simulink model "T2_DCACpart_solar"  (R2022b)
settings: Solver=VariableStepAuto  StartTime=0.0  StopTime=10.0  RelTol=1e-3
undefined symbols (not defined in the file): High, Low, Ts
libraries: fl_lib x94, nesl_utility x50, simulink x14, ee_lib x2
(part 1 of 2)
settings Model: Creator=mingreico  LastModifiedBy=mingreico

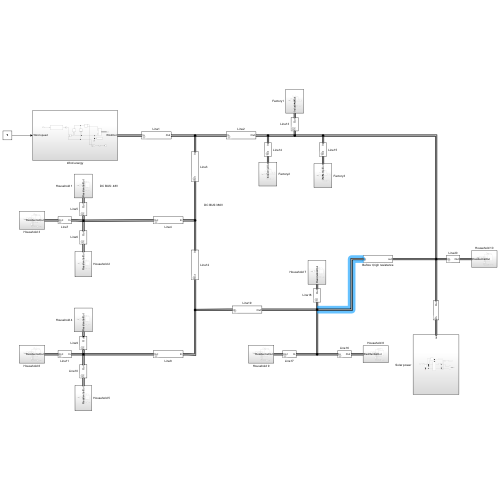
[thumbnail: Simulink's stored preview of the top-level diagram]
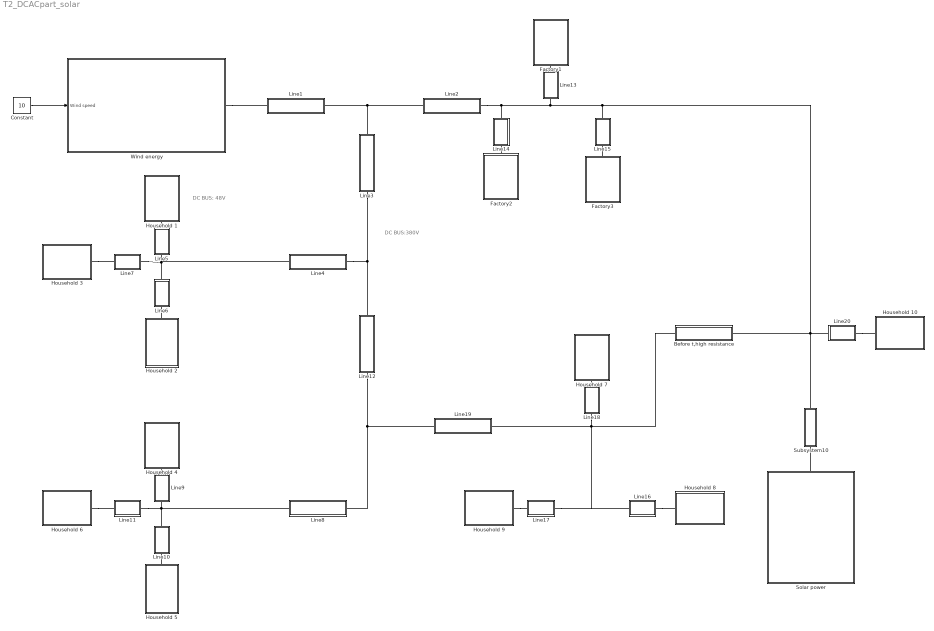
== system T2_DCACpart_solar ==
  note: DC BUS: 48V
  note: DC BUS:380V
  Before t,high resistance : Subsystem  mask{t=48}
      mask prompts: t "Specific jumping time"
  Constant : Constant  Value=10
  Factory1 : Subsystem
  Factory2 : Subsystem
  Factory3 : Subsystem
  Household 1 : Subsystem
  Household 10 : Subsystem
  Household 2 : Subsystem
  Household 3 : Subsystem
  Household 4 : Subsystem
  Household 5 : Subsystem
  Household 6 : Subsystem
  Household 7 : Subsystem
  Household 8 : Subsystem
  Household 9 : Subsystem
  Line1 : Subsystem  mask{rho=1.68e-8, l=2.0, A=1.5e-6}
      mask prompts: rho "Specific resistivity in Ohm*m"; l "Length in m"; A "Cross sectional area in m^2"
  Line10 : Subsystem  mask{rho=1.68e-8, l=2.0, A=1.5e-6}
      mask prompts: rho "Specific resistivity in Ohm*m"; l "Length in m"; A "Cross sectional area in m^2"
  Line11 : Subsystem  mask{rho=1.68e-8, l=2.0, A=1.5e-6}
      mask prompts: rho "Specific resistivity in Ohm*m"; l "Length in m"; A "Cross sectional area in m^2"
  Line12 : Subsystem  mask{rho=1.68e-8, l=2.0, A=1.5e-6}
      mask prompts: rho "Specific resistivity in Ohm*m"; l "Length in m"; A "Cross sectional area in m^2"
  Line13 : Subsystem  mask{rho=1.68e-8, l=2.0, A=1.5e-6}
      mask prompts: rho "Specific resistivity in Ohm*m"; l "Length in m"; A "Cross sectional area in m^2"
  Line14 : Subsystem  mask{rho=1.68e-8, l=2.0, A=1.5e-6}
      mask prompts: rho "Specific resistivity in Ohm*m"; l "Length in m"; A "Cross sectional area in m^2"
  Line15 : Subsystem  mask{rho=1.68e-8, l=2.0, A=1.5e-6}
      mask prompts: rho "Specific resistivity in Ohm*m"; l "Length in m"; A "Cross sectional area in m^2"
  Line16 : Subsystem  mask{rho=1.68e-8, l=2.0, A=1.5e-6}
      mask prompts: rho "Specific resistivity in Ohm*m"; l "Length in m"; A "Cross sectional area in m^2"
  Line17 : Subsystem  mask{rho=1.68e-8, l=2.0, A=1.5e-6}
      mask prompts: rho "Specific resistivity in Ohm*m"; l "Length in m"; A "Cross sectional area in m^2"
  Line18 : Subsystem  mask{rho=1.68e-8, l=2.0, A=1.5e-6}
      mask prompts: rho "Specific resistivity in Ohm*m"; l "Length in m"; A "Cross sectional area in m^2"
  Line19 : Subsystem  mask{rho=1.68e-8, l=2.0, A=1.5e-6}
      mask prompts: rho "Specific resistivity in Ohm*m"; l "Length in m"; A "Cross sectional area in m^2"
  Line2 : Subsystem  mask{rho=1.68e-8, l=2.0, A=1.5e-6}
      mask prompts: rho "Specific resistivity in Ohm*m"; l "Length in m"; A "Cross sectional area in m^2"
  Line20 : Subsystem  mask{rho=1.68e-8, l=2.0, A=1.5e-6}
      mask prompts: rho "Specific resistivity in Ohm*m"; l "Length in m"; A "Cross sectional area in m^2"
  Line3 : Subsystem  mask{rho=1.68e-8, l=2.0, A=1.5e-6}
      mask prompts: rho "Specific resistivity in Ohm*m"; l "Length in m"; A "Cross sectional area in m^2"
  Line4 : Subsystem  mask{rho=1.68e-8, l=2.0, A=1.5e-6}
      mask prompts: rho "Specific resistivity in Ohm*m"; l "Length in m"; A "Cross sectional area in m^2"
  Line5 : Subsystem  mask{rho=1.68e-8, l=2.0, A=1.5e-6}
      mask prompts: rho "Specific resistivity in Ohm*m"; l "Length in m"; A "Cross sectional area in m^2"
  Line6 : Subsystem  mask{rho=1.68e-8, l=2.0, A=1.5e-6}
      mask prompts: rho "Specific resistivity in Ohm*m"; l "Length in m"; A "Cross sectional area in m^2"
  Line7 : Subsystem  mask{rho=1.68e-8, l=2.0, A=1.5e-6}
      mask prompts: rho "Specific resistivity in Ohm*m"; l "Length in m"; A "Cross sectional area in m^2"
  Line8 : Subsystem  mask{rho=1.68e-8, l=2.0, A=1.5e-6}
      mask prompts: rho "Specific resistivity in Ohm*m"; l "Length in m"; A "Cross sectional area in m^2"
  Line9 : Subsystem  mask{rho=1.68e-8, l=2.0, A=1.5e-6}
      mask prompts: rho "Specific resistivity in Ohm*m"; l "Length in m"; A "Cross sectional area in m^2"
  Solar power : Subsystem
  Subsystem10 : Subsystem  mask{rho=1.68e-8, l=2.0, A=1.5e-6}
      mask prompts: rho "Specific resistivity in Ohm*m"; l "Length in m"; A "Cross sectional area in m^2"
  Wind energy : Subsystem
  wires:
  Constant/1 -> Wind energy/1(Wind speed)
  connections:
  Wind energy/RConn1 -- Line1/LConn1
  Line2/LConn1 -- Line3/LConn1 -- Line1/RConn1
  Household 1/RConn1 -- Line5/RConn1
  Household 3/RConn1 -- Line7/RConn1
  Household 2/RConn1 -- Line6/LConn1
  Line5/LConn1 -- Line6/RConn1 -- Line7/LConn1 -- Line4/RConn1
  Line9/LConn1 -- Line11/LConn1 -- Line10/RConn1 -- Line8/RConn1
  Household 5/RConn1 -- Line10/LConn1
  Household 6/RConn1 -- Line11/RConn1
  Household 4/RConn1 -- Line9/RConn1
  Line3/RConn1 -- Line4/LConn1 -- Line12/LConn1
  Line12/RConn1 -- Line19/LConn1 -- Line8/LConn1
  Line2/RConn1 -- Line14/LConn1 -- Line13/LConn1 -- Before t,high resistance/RConn1 -- Line20/LConn1 -- Subsystem10/RConn1 -- Line15/LConn1
  Factory1/RConn1 -- Line13/RConn1
  Factory2/RConn1 -- Line14/RConn1
  Factory3/RConn1 -- Line15/RConn1
  Household 9/RConn1 -- Line17/RConn1
  Household 7/RConn1 -- Line18/RConn1
  Line18/LConn1 -- Before t,high resistance/LConn1 -- Line16/LConn1 -- Line17/LConn1 -- Line19/RConn1
  Line16/RConn1 -- Household 8/RConn1
  Line20/RConn1 -- Household 10/RConn1
  Solar power/LConn1 -- Subsystem10/LConn1

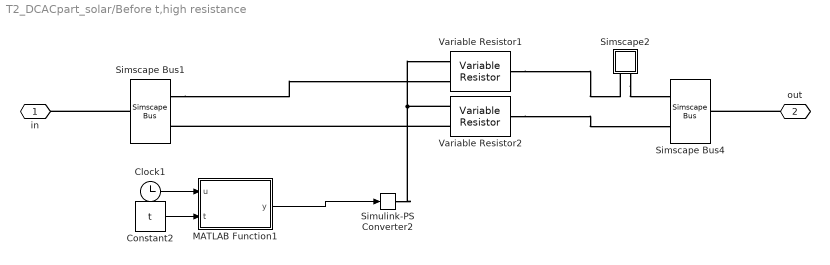
== system T2_DCACpart_solar/Before t,high resistance ==
  Clock1 : Clock
  Constant2 : Constant  Value=t
  MATLAB Function1 : MATLAB Function  TreatAsAtomicUnit=on
  Simscape Bus1 : SimscapeBus  HierarchyStrings=High;Low
  Simscape Bus4 : SimscapeBus  HierarchyStrings=High;Low
  Simscape2 : Subsystem
      mask Display:
      | disp('A')
      | port_label('LConn',1,'+')
      | port_label('LConn',2,'-')
  Simulink-PS Converter2 : nesl_utility/Simulink-PS Converter  PhysicalDomain=network_engine_domain  SubClassName=ps_input  LeftPortType=input  RightPortType=output  PseudoPeriodic=off  Frequencies=[]  NoiseDistribution=none  NoiseParameters=[]  Unit=1  AffineConversion=off  FilteringAndDerivatives=provide  SimscapeFilterOrder=1  InputFilterTimeConstant=0.001  UdotUserProvided=0
  Variable Resistor1 : fl_lib/Electrical/Electrical Elements/Variable Resistor  Rmin=0 Ohm  i_specify=off  i_priority=None  i=0 A  i_nominal_specify=off  i_nominal_unit=A  i_nominal_value=1  v_specify=off  v_priority=None  v=0 V  v_nominal_specify=off  v_nominal_unit=V  v_nominal_value=1
  Variable Resistor2 : fl_lib/Electrical/Electrical Elements/Variable Resistor  Rmin=0 Ohm  i_specify=off  i_priority=None  i=0 A  i_nominal_specify=off  i_nominal_unit=A  i_nominal_value=1  v_specify=off  v_priority=None  v=0 V  v_nominal_specify=off  v_nominal_unit=V  v_nominal_value=1
  in : PMIOPort  Side=Left
  out : PMIOPort  Port=2  Side=Right
  wires:
  MATLAB Function1/1(y) -> Simulink-PS Converter2/1
  Constant2/1 -> MATLAB Function1/2(t)
  Clock1/1 -> MATLAB Function1/1(u)
  connections:
  out/RConn1 -- Simscape Bus4/RConn1
  Simscape Bus1/RConn1 -- in/RConn1
  Variable Resistor2/LConn2 -- Simscape Bus1/LConn2
  Simscape Bus1/LConn1 -- Variable Resistor1/LConn2
  Variable Resistor1/RConn1 -- Simscape2/LConn1
  Variable Resistor2/RConn1 -- Simscape Bus4/LConn2
  Simulink-PS Converter2/RConn1 -- Variable Resistor2/LConn1 -- Variable Resistor1/LConn1
  Simscape2/LConn2 -- Simscape Bus4/LConn1

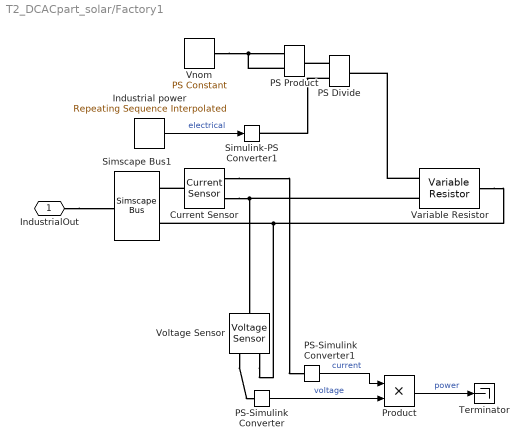
== system T2_DCACpart_solar/Factory1 ==
  Current Sensor : fl_lib/Electrical/Electrical Sensors/Current Sensor
  "Industrial power " : simulink/Sources/Repeating Sequence Interpolated  OutValues=[6.0 5.9 5.9 5.9 5.8 5.7 5.6 5.5 5.7 5.9 5.9 5.3 5.3 5.6 5.9 5.8 5.6 5.3 5.3 5.7 5.9 5.9 6.0 6.0]*1000  TimeValues=[0 1 2 3 4 5 6 7 8 9 10 11 12 13 14 15 16 17 18 19 20 21 22 23]  LookUpMeth=Interpolation-Use End Values  tsamp=1e-4  OutMin=[]  OutMax=[]  OutDataTypeStr=double  OutputDataTypeScalingMode=double  OutDataType=fixdt(0,8)  OutScaling=2^-10
  PS Divide : fl_lib/Physical Signals/Functions/PS Divide
  PS Product : fl_lib/Physical Signals/Functions/PS Product
  PS-Simulink Converter : nesl_utility/PS-Simulink Converter  PhysicalDomain=network_engine_domain  SubClassName=ps_output  LeftPortType=input  RightPortType=output  PseudoPeriodic=off  Frequencies=[]  VectorFormat=inherit  Unit=inherit  AffineConversion=off
  PS-Simulink Converter1 : nesl_utility/PS-Simulink Converter  PhysicalDomain=network_engine_domain  SubClassName=ps_output  LeftPortType=input  RightPortType=output  PseudoPeriodic=off  Frequencies=[]  VectorFormat=inherit  Unit=inherit  AffineConversion=off
  Product : Product
  Simscape Bus1 : SimscapeBus  HierarchyStrings=High;Low
  Simulink-PS Converter1 : nesl_utility/Simulink-PS Converter  PhysicalDomain=network_engine_domain  SubClassName=ps_input  LeftPortType=input  RightPortType=output  PseudoPeriodic=off  Frequencies=[]  NoiseDistribution=none  NoiseParameters=[]  Unit=V*A  AffineConversion=off  FilteringAndDerivatives=provide  SimscapeFilterOrder=1  InputFilterTimeConstant=0.001  UdotUserProvided=0
  Terminator : Terminator
  Variable Resistor : fl_lib/Electrical/Electrical Elements/Variable Resistor  Rmin=0 Ohm  i_specify=off  i_priority=None  i=0 A  i_nominal_specify=off  i_nominal_unit=A  i_nominal_value=1  v_specify=off  v_priority=None  v=0 V  v_nominal_specify=off  v_nominal_unit=V  v_nominal_value=1
  Vnom : fl_lib/Physical Signals/Sources/PS Constant  constant=48 V
  Voltage Sensor : fl_lib/Electrical/Electrical Sensors/Voltage Sensor
  IndustrialOut : PMIOPort  Side=Right
  wires:
  Product/1 -> Terminator/1  "power"
  PS-Simulink Converter1/1 -> Product/1  "current"
  PS-Simulink Converter/1 -> Product/2  "voltage"
  "Industrial power "/1 -> Simulink-PS Converter1/1  "electrical"
  connections:
  Current Sensor/RConn1 -- PS-Simulink Converter1/LConn1
  Current Sensor/LConn1 -- Simscape Bus1/LConn1
  Voltage Sensor/RConn1 -- PS-Simulink Converter/LConn1
  Current Sensor/RConn2 -- Variable Resistor/LConn2 -- Voltage Sensor/LConn1
  IndustrialOut/RConn1 -- Simscape Bus1/RConn1
  Voltage Sensor/RConn2 -- Simscape Bus1/LConn2 -- Variable Resistor/RConn1
  Vnom/RConn1 -- PS Product/LConn2 -- PS Product/LConn1
  PS Divide/LConn2 -- Simulink-PS Converter1/RConn1
  Variable Resistor/LConn1 -- PS Divide/RConn1
  PS Divide/LConn1 -- PS Product/RConn1

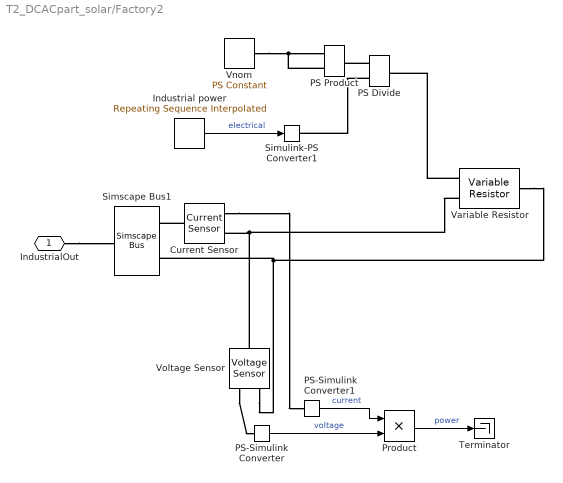
== system T2_DCACpart_solar/Factory2 ==
  Current Sensor : fl_lib/Electrical/Electrical Sensors/Current Sensor
  "Industrial power " : simulink/Sources/Repeating Sequence Interpolated  OutValues=[6.0 5.9 5.9 5.9 5.8 5.7 5.6 5.5 5.7 5.9 5.9 5.3 5.3 5.6 5.9 5.8 5.6 5.3 5.3 5.7 5.9 5.9 6.0 6.0]*1000  TimeValues=[0 1 2 3 4 5 6 7 8 9 10 11 12 13 14 15 16 17 18 19 20 21 22 23]  LookUpMeth=Interpolation-Use End Values  tsamp=1e-4  OutMin=[]  OutMax=[]  OutDataTypeStr=double  OutputDataTypeScalingMode=double  OutDataType=fixdt(0,8)  OutScaling=2^-10
  PS Divide : fl_lib/Physical Signals/Functions/PS Divide
  PS Product : fl_lib/Physical Signals/Functions/PS Product
  PS-Simulink Converter : nesl_utility/PS-Simulink Converter  PhysicalDomain=network_engine_domain  SubClassName=ps_output  LeftPortType=input  RightPortType=output  PseudoPeriodic=off  Frequencies=[]  VectorFormat=inherit  Unit=inherit  AffineConversion=off
  PS-Simulink Converter1 : nesl_utility/PS-Simulink Converter  PhysicalDomain=network_engine_domain  SubClassName=ps_output  LeftPortType=input  RightPortType=output  PseudoPeriodic=off  Frequencies=[]  VectorFormat=inherit  Unit=inherit  AffineConversion=off
  Product : Product
  Simscape Bus1 : SimscapeBus  HierarchyStrings=High;Low
  Simulink-PS Converter1 : nesl_utility/Simulink-PS Converter  PhysicalDomain=network_engine_domain  SubClassName=ps_input  LeftPortType=input  RightPortType=output  PseudoPeriodic=off  Frequencies=[]  NoiseDistribution=none  NoiseParameters=[]  Unit=V*A  AffineConversion=off  FilteringAndDerivatives=provide  SimscapeFilterOrder=1  InputFilterTimeConstant=0.001  UdotUserProvided=0
  Terminator : Terminator
  Variable Resistor : fl_lib/Electrical/Electrical Elements/Variable Resistor  Rmin=0 Ohm  i_specify=off  i_priority=None  i=0 A  i_nominal_specify=off  i_nominal_unit=A  i_nominal_value=1  v_specify=off  v_priority=None  v=0 V  v_nominal_specify=off  v_nominal_unit=V  v_nominal_value=1
  Vnom : fl_lib/Physical Signals/Sources/PS Constant  constant=48 V
  Voltage Sensor : fl_lib/Electrical/Electrical Sensors/Voltage Sensor
  IndustrialOut : PMIOPort  Side=Right
  wires:
  PS-Simulink Converter/1 -> Product/2  "voltage"
  PS-Simulink Converter1/1 -> Product/1  "current"
  Product/1 -> Terminator/1  "power"
  "Industrial power "/1 -> Simulink-PS Converter1/1  "electrical"
  connections:
  Voltage Sensor/RConn2 -- Variable Resistor/RConn1 -- Simscape Bus1/LConn2
  IndustrialOut/RConn1 -- Simscape Bus1/RConn1
  Voltage Sensor/LConn1 -- Variable Resistor/LConn2 -- Current Sensor/RConn2
  Voltage Sensor/RConn1 -- PS-Simulink Converter/LConn1
  Current Sensor/LConn1 -- Simscape Bus1/LConn1
  Current Sensor/RConn1 -- PS-Simulink Converter1/LConn1
  Vnom/RConn1 -- PS Product/LConn2 -- PS Product/LConn1
  Variable Resistor/LConn1 -- PS Divide/RConn1
  PS Divide/LConn1 -- PS Product/RConn1
  PS Divide/LConn2 -- Simulink-PS Converter1/RConn1

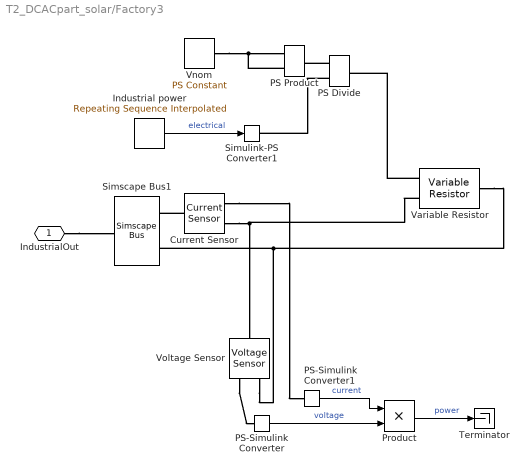
== system T2_DCACpart_solar/Factory3 ==
  Current Sensor : fl_lib/Electrical/Electrical Sensors/Current Sensor
  "Industrial power " : simulink/Sources/Repeating Sequence Interpolated  OutValues=[6.0 5.9 5.9 5.9 5.8 5.7 5.6 5.5 5.7 5.9 5.9 5.3 5.3 5.6 5.9 5.8 5.6 5.3 5.3 5.7 5.9 5.9 6.0 6.0]*1000  TimeValues=[0 1 2 3 4 5 6 7 8 9 10 11 12 13 14 15 16 17 18 19 20 21 22 23]  LookUpMeth=Interpolation-Use End Values  tsamp=1e-4  OutMin=[]  OutMax=[]  OutDataTypeStr=double  OutputDataTypeScalingMode=double  OutDataType=fixdt(0,8)  OutScaling=2^-10
  PS Divide : fl_lib/Physical Signals/Functions/PS Divide
  PS Product : fl_lib/Physical Signals/Functions/PS Product
  PS-Simulink Converter : nesl_utility/PS-Simulink Converter  PhysicalDomain=network_engine_domain  SubClassName=ps_output  LeftPortType=input  RightPortType=output  PseudoPeriodic=off  Frequencies=[]  VectorFormat=inherit  Unit=inherit  AffineConversion=off
  PS-Simulink Converter1 : nesl_utility/PS-Simulink Converter  PhysicalDomain=network_engine_domain  SubClassName=ps_output  LeftPortType=input  RightPortType=output  PseudoPeriodic=off  Frequencies=[]  VectorFormat=inherit  Unit=inherit  AffineConversion=off
  Product : Product
  Simscape Bus1 : SimscapeBus  HierarchyStrings=High;Low
  Simulink-PS Converter1 : nesl_utility/Simulink-PS Converter  PhysicalDomain=network_engine_domain  SubClassName=ps_input  LeftPortType=input  RightPortType=output  PseudoPeriodic=off  Frequencies=[]  NoiseDistribution=none  NoiseParameters=[]  Unit=V*A  AffineConversion=off  FilteringAndDerivatives=provide  SimscapeFilterOrder=1  InputFilterTimeConstant=0.001  UdotUserProvided=0
  Terminator : Terminator
  Variable Resistor : fl_lib/Electrical/Electrical Elements/Variable Resistor  Rmin=0 Ohm  i_specify=off  i_priority=None  i=0 A  i_nominal_specify=off  i_nominal_unit=A  i_nominal_value=1  v_specify=off  v_priority=None  v=0 V  v_nominal_specify=off  v_nominal_unit=V  v_nominal_value=1
  Vnom : fl_lib/Physical Signals/Sources/PS Constant  constant=48 V
  Voltage Sensor : fl_lib/Electrical/Electrical Sensors/Voltage Sensor
  IndustrialOut : PMIOPort  Side=Right
  wires:
  Product/1 -> Terminator/1  "power"
  PS-Simulink Converter1/1 -> Product/1  "current"
  PS-Simulink Converter/1 -> Product/2  "voltage"
  "Industrial power "/1 -> Simulink-PS Converter1/1  "electrical"
  connections:
  Current Sensor/RConn1 -- PS-Simulink Converter1/LConn1
  Current Sensor/LConn1 -- Simscape Bus1/LConn1
  Voltage Sensor/RConn1 -- PS-Simulink Converter/LConn1
  Current Sensor/RConn2 -- Variable Resistor/LConn2 -- Voltage Sensor/LConn1
  IndustrialOut/RConn1 -- Simscape Bus1/RConn1
  Voltage Sensor/RConn2 -- Simscape Bus1/LConn2 -- Variable Resistor/RConn1
  Vnom/RConn1 -- PS Product/LConn2 -- PS Product/LConn1
  Variable Resistor/LConn1 -- PS Divide/RConn1
  PS Divide/LConn1 -- PS Product/RConn1
  PS Divide/LConn2 -- Simulink-PS Converter1/RConn1

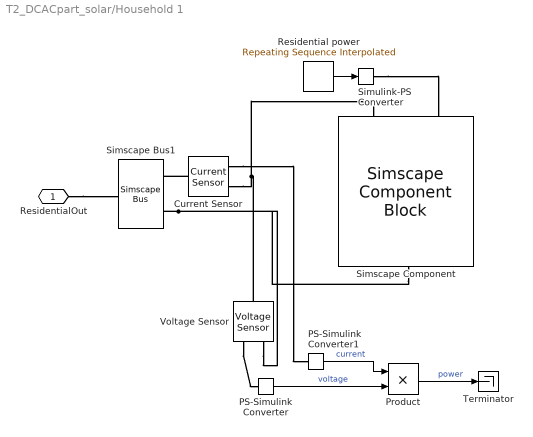
== system T2_DCACpart_solar/Household 1 ==
  Current Sensor : fl_lib/Electrical/Electrical Sensors/Current Sensor
  PS-Simulink Converter : nesl_utility/PS-Simulink Converter  PhysicalDomain=network_engine_domain  SubClassName=ps_output  LeftPortType=input  RightPortType=output  PseudoPeriodic=off  Frequencies=[]  VectorFormat=inherit  Unit=inherit  AffineConversion=off
  PS-Simulink Converter1 : nesl_utility/PS-Simulink Converter  PhysicalDomain=network_engine_domain  SubClassName=ps_output  LeftPortType=input  RightPortType=output  PseudoPeriodic=off  Frequencies=[]  VectorFormat=inherit  Unit=inherit  AffineConversion=off
  Product : Product
  "Residential power " : simulink/Sources/Repeating Sequence Interpolated  OutValues=[2.8 2.5 2 2 2.2 2.5 2.8 3.4 3.6 3.8 4 4 4 4 4 4 4 4 4 4 3.8 3.5 3.2 3]*1000  TimeValues=[0 1 2 3 4 5 6 7 8 9 10 11 12 13 14 15 16 17 18 19 20 21 22 23]  LookUpMeth=Interpolation-Use End Values  tsamp=1e-4  OutMin=[]  OutMax=[]  OutDataTypeStr=double  OutputDataTypeScalingMode=double  OutDataType=fixdt(0,8)  OutScaling=2^-10
  Simscape Component : SimscapeComponentBlock  SourceFile=ResidentialPowerLoad  ComponentPath=ResidentialPowerLoad  ComponentVariants="[\"ResidentialPowerLoad\"]"  ComponentVariantNames="[\"ResidentialPowerLoad\"]"  ClassName=ResidentialPowerLoad  SchemaVersion=1  i_specify=off  i_priority=None  i=0 A  i_nominal_specify=off  i_nominal_unit=A  i_nominal_value=1  v_specify=off  v_priority=None  v=0 V  v_nominal_specify=off  v_nominal_unit=V  v_nominal_value=1
      settings: CopyFcn=simscape.engine.sli.internal.componentblockcallback(gcbh,'COPY')  PreCopyFcn=simscape.engine.sli.internal.componentblockcallback(gcbh,'PRECOPY')  PreDeleteFcn=simscape.engine.sli.internal.componentblockcallback(gcbh,'PREDELETE')  InternalSimscapePortConfiguration="{\"Bottom\":[],\"Left\":[{\"id\":\"Power\",\"label\":\"P\",\"type\":\"input\"},{\"id\":\"p\",\"label\":\"+\",\"type\":\"foundation.electrical.electrical\"}],\"Right\":[{\"id\":\"n\",\"label\":\"-\",\"type\":\"foundation.electrical.electrical\"}],\"Top\":[]}"
      mask Type: ResidentialPowerLoad
      mask Display: color('red');plot([0 1 1 0 0],[0 0 1 1 0]);plot([0.7,1],[1,0.7]);plot(-2,-1.75);plot(3, 1);disp('\n.ssc\nUnresolved')
  Simscape Bus1 : SimscapeBus  HierarchyStrings=High;Low
  Simulink-PS Converter : nesl_utility/Simulink-PS Converter  PhysicalDomain=network_engine_domain  SubClassName=ps_input  LeftPortType=input  RightPortType=output  PseudoPeriodic=off  Frequencies=[]  NoiseDistribution=none  NoiseParameters=[]  Unit=1  AffineConversion=off  FilteringAndDerivatives=provide  SimscapeFilterOrder=1  InputFilterTimeConstant=0.001  UdotUserProvided=0
  Terminator : Terminator
  Voltage Sensor : fl_lib/Electrical/Electrical Sensors/Voltage Sensor
  ResidentialOut : PMIOPort  Side=Right
  wires:
  "Residential power "/1 -> Simulink-PS Converter/1
  PS-Simulink Converter/1 -> Product/2  "voltage"
  PS-Simulink Converter1/1 -> Product/1  "current"
  Product/1 -> Terminator/1  "power"
  connections:
  Simscape Bus1/LConn2 -- Simscape Component/RConn1 -- Voltage Sensor/RConn2
  ResidentialOut/RConn1 -- Simscape Bus1/RConn1
  Current Sensor/RConn2 -- Voltage Sensor/LConn1 -- Simscape Component/LConn2
  Voltage Sensor/RConn1 -- PS-Simulink Converter/LConn1
  Simulink-PS Converter/RConn1 -- Simscape Component/LConn1
  Current Sensor/LConn1 -- Simscape Bus1/LConn1
  Current Sensor/RConn1 -- PS-Simulink Converter1/LConn1

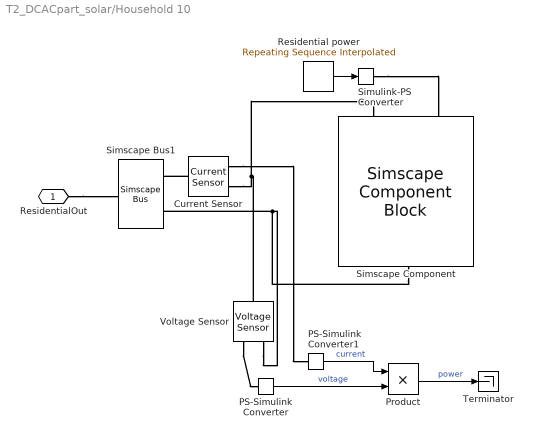
== system T2_DCACpart_solar/Household 10 ==
  Current Sensor : fl_lib/Electrical/Electrical Sensors/Current Sensor
  PS-Simulink Converter : nesl_utility/PS-Simulink Converter  PhysicalDomain=network_engine_domain  SubClassName=ps_output  LeftPortType=input  RightPortType=output  PseudoPeriodic=off  Frequencies=[]  VectorFormat=inherit  Unit=inherit  AffineConversion=off
  PS-Simulink Converter1 : nesl_utility/PS-Simulink Converter  PhysicalDomain=network_engine_domain  SubClassName=ps_output  LeftPortType=input  RightPortType=output  PseudoPeriodic=off  Frequencies=[]  VectorFormat=inherit  Unit=inherit  AffineConversion=off
  Product : Product
  "Residential power " : simulink/Sources/Repeating Sequence Interpolated  OutValues=[2.8 2.5 2 2 2.2 2.5 2.8 3.4 3.6 3.8 4 4 4 4 4 4 4 4 4 4 3.8 3.5 3.2 3]*1000  TimeValues=[0 1 2 3 4 5 6 7 8 9 10 11 12 13 14 15 16 17 18 19 20 21 22 23]  LookUpMeth=Interpolation-Use End Values  tsamp=1e-4  OutMin=[]  OutMax=[]  OutDataTypeStr=double  OutputDataTypeScalingMode=double  OutDataType=fixdt(0,8)  OutScaling=2^-10
  Simscape Component : SimscapeComponentBlock  SourceFile=ResidentialPowerLoad  ComponentPath=ResidentialPowerLoad  ComponentVariants="[\"ResidentialPowerLoad\"]"  ComponentVariantNames="[\"ResidentialPowerLoad\"]"  ClassName=ResidentialPowerLoad  SchemaVersion=1  i_specify=off  i_priority=None  i=0 A  i_nominal_specify=off  i_nominal_unit=A  i_nominal_value=1  v_specify=off  v_priority=None  v=0 V  v_nominal_specify=off  v_nominal_unit=V  v_nominal_value=1
      settings: CopyFcn=simscape.engine.sli.internal.componentblockcallback(gcbh,'COPY')  PreCopyFcn=simscape.engine.sli.internal.componentblockcallback(gcbh,'PRECOPY')  PreDeleteFcn=simscape.engine.sli.internal.componentblockcallback(gcbh,'PREDELETE')  InternalSimscapePortConfiguration="{\"Bottom\":[],\"Left\":[{\"id\":\"Power\",\"label\":\"P\",\"type\":\"input\"},{\"id\":\"p\",\"label\":\"+\",\"type\":\"foundation.electrical.electrical\"}],\"Right\":[{\"id\":\"n\",\"label\":\"-\",\"type\":\"foundation.electrical.electrical\"}],\"Top\":[]}"
      mask Type: ResidentialPowerLoad
      mask Display: color('red');plot([0 1 1 0 0],[0 0 1 1 0]);plot([0.7,1],[1,0.7]);plot(-2,-1.75);plot(3, 1);disp('\n.ssc\nUnresolved')
  Simscape Bus1 : SimscapeBus  HierarchyStrings=High;Low
  Simulink-PS Converter : nesl_utility/Simulink-PS Converter  PhysicalDomain=network_engine_domain  SubClassName=ps_input  LeftPortType=input  RightPortType=output  PseudoPeriodic=off  Frequencies=[]  NoiseDistribution=none  NoiseParameters=[]  Unit=1  AffineConversion=off  FilteringAndDerivatives=provide  SimscapeFilterOrder=1  InputFilterTimeConstant=0.001  UdotUserProvided=0
  Terminator : Terminator
  Voltage Sensor : fl_lib/Electrical/Electrical Sensors/Voltage Sensor
  ResidentialOut : PMIOPort  Side=Right
  wires:
  Product/1 -> Terminator/1  "power"
  PS-Simulink Converter1/1 -> Product/1  "current"
  PS-Simulink Converter/1 -> Product/2  "voltage"
  "Residential power "/1 -> Simulink-PS Converter/1
  connections:
  Current Sensor/RConn1 -- PS-Simulink Converter1/LConn1
  Current Sensor/LConn1 -- Simscape Bus1/LConn1
  Simulink-PS Converter/RConn1 -- Simscape Component/LConn1
  Voltage Sensor/RConn1 -- PS-Simulink Converter/LConn1
  Voltage Sensor/LConn1 -- Current Sensor/RConn2 -- Simscape Component/LConn2
  ResidentialOut/RConn1 -- Simscape Bus1/RConn1
  Simscape Component/RConn1 -- Simscape Bus1/LConn2 -- Voltage Sensor/RConn2

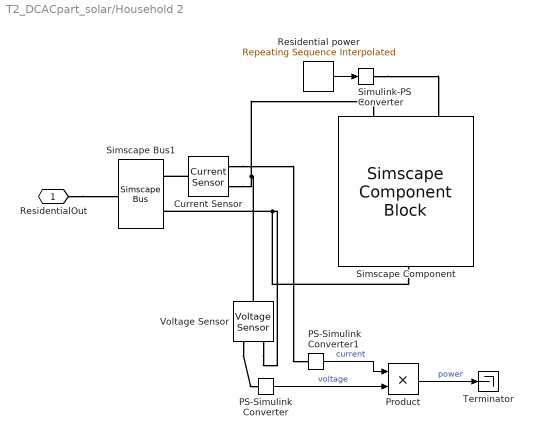
== system T2_DCACpart_solar/Household 2 ==
  Current Sensor : fl_lib/Electrical/Electrical Sensors/Current Sensor
  PS-Simulink Converter : nesl_utility/PS-Simulink Converter  PhysicalDomain=network_engine_domain  SubClassName=ps_output  LeftPortType=input  RightPortType=output  PseudoPeriodic=off  Frequencies=[]  VectorFormat=inherit  Unit=inherit  AffineConversion=off
  PS-Simulink Converter1 : nesl_utility/PS-Simulink Converter  PhysicalDomain=network_engine_domain  SubClassName=ps_output  LeftPortType=input  RightPortType=output  PseudoPeriodic=off  Frequencies=[]  VectorFormat=inherit  Unit=inherit  AffineConversion=off
  Product : Product
  "Residential power " : simulink/Sources/Repeating Sequence Interpolated  OutValues=[2.8 2.5 2 2 2.2 2.5 2.8 3.4 3.6 3.8 4 4 4 4 4 4 4 4 4 4 3.8 3.5 3.2 3]*1000  TimeValues=[0 1 2 3 4 5 6 7 8 9 10 11 12 13 14 15 16 17 18 19 20 21 22 23]  LookUpMeth=Interpolation-Use End Values  tsamp=1e-4  OutMin=[]  OutMax=[]  OutDataTypeStr=double  OutputDataTypeScalingMode=double  OutDataType=fixdt(0,8)  OutScaling=2^-10
  Simscape Component : SimscapeComponentBlock  SourceFile=ResidentialPowerLoad  ComponentPath=ResidentialPowerLoad  ComponentVariants="[\"ResidentialPowerLoad\"]"  ComponentVariantNames="[\"ResidentialPowerLoad\"]"  ClassName=ResidentialPowerLoad  SchemaVersion=1  i_specify=off  i_priority=None  i=0 A  i_nominal_specify=off  i_nominal_unit=A  i_nominal_value=1  v_specify=off  v_priority=None  v=0 V  v_nominal_specify=off  v_nominal_unit=V  v_nominal_value=1
      settings: CopyFcn=simscape.engine.sli.internal.componentblockcallback(gcbh,'COPY')  PreCopyFcn=simscape.engine.sli.internal.componentblockcallback(gcbh,'PRECOPY')  PreDeleteFcn=simscape.engine.sli.internal.componentblockcallback(gcbh,'PREDELETE')  InternalSimscapePortConfiguration="{\"Bottom\":[],\"Left\":[{\"id\":\"Power\",\"label\":\"P\",\"type\":\"input\"},{\"id\":\"p\",\"label\":\"+\",\"type\":\"foundation.electrical.electrical\"}],\"Right\":[{\"id\":\"n\",\"label\":\"-\",\"type\":\"foundation.electrical.electrical\"}],\"Top\":[]}"
      mask Type: ResidentialPowerLoad
      mask Display: color('red');plot([0 1 1 0 0],[0 0 1 1 0]);plot([0.7,1],[1,0.7]);plot(-2,-1.75);plot(3, 1);disp('\n.ssc\nUnresolved')
  Simscape Bus1 : SimscapeBus  HierarchyStrings=High;Low
  Simulink-PS Converter : nesl_utility/Simulink-PS Converter  PhysicalDomain=network_engine_domain  SubClassName=ps_input  LeftPortType=input  RightPortType=output  PseudoPeriodic=off  Frequencies=[]  NoiseDistribution=none  NoiseParameters=[]  Unit=1  AffineConversion=off  FilteringAndDerivatives=provide  SimscapeFilterOrder=1  InputFilterTimeConstant=0.001  UdotUserProvided=0
  Terminator : Terminator
  Voltage Sensor : fl_lib/Electrical/Electrical Sensors/Voltage Sensor
  ResidentialOut : PMIOPort  Side=Right
  wires:
  Product/1 -> Terminator/1  "power"
  PS-Simulink Converter1/1 -> Product/1  "current"
  PS-Simulink Converter/1 -> Product/2  "voltage"
  "Residential power "/1 -> Simulink-PS Converter/1
  connections:
  Current Sensor/RConn1 -- PS-Simulink Converter1/LConn1
  Current Sensor/LConn1 -- Simscape Bus1/LConn1
  Simulink-PS Converter/RConn1 -- Simscape Component/LConn1
  Voltage Sensor/RConn1 -- PS-Simulink Converter/LConn1
  Voltage Sensor/LConn1 -- Current Sensor/RConn2 -- Simscape Component/LConn2
  ResidentialOut/RConn1 -- Simscape Bus1/RConn1
  Simscape Component/RConn1 -- Simscape Bus1/LConn2 -- Voltage Sensor/RConn2

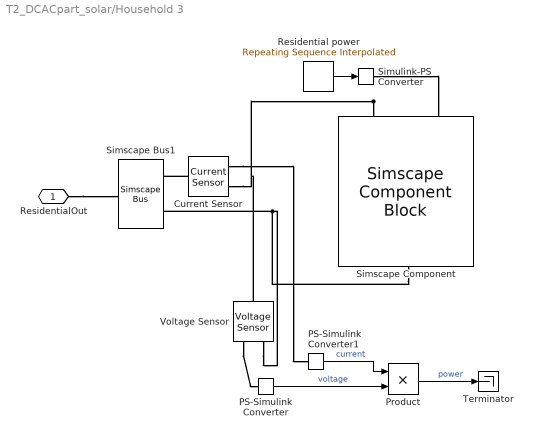
== system T2_DCACpart_solar/Household 3 ==
  Current Sensor : fl_lib/Electrical/Electrical Sensors/Current Sensor
  PS-Simulink Converter : nesl_utility/PS-Simulink Converter  PhysicalDomain=network_engine_domain  SubClassName=ps_output  LeftPortType=input  RightPortType=output  PseudoPeriodic=off  Frequencies=[]  VectorFormat=inherit  Unit=inherit  AffineConversion=off
  PS-Simulink Converter1 : nesl_utility/PS-Simulink Converter  PhysicalDomain=network_engine_domain  SubClassName=ps_output  LeftPortType=input  RightPortType=output  PseudoPeriodic=off  Frequencies=[]  VectorFormat=inherit  Unit=inherit  AffineConversion=off
  Product : Product
  "Residential power " : simulink/Sources/Repeating Sequence Interpolated  OutValues=[2.8 2.5 2 2 2.2 2.5 2.8 3.4 3.6 3.8 4 4 4 4 4 4 4 4 4 4 3.8 3.5 3.2 3]*1000  TimeValues=[0 1 2 3 4 5 6 7 8 9 10 11 12 13 14 15 16 17 18 19 20 21 22 23]  LookUpMeth=Interpolation-Use End Values  tsamp=1e-4  OutMin=[]  OutMax=[]  OutDataTypeStr=double  OutputDataTypeScalingMode=double  OutDataType=fixdt(0,8)  OutScaling=2^-10
  Simscape Component : SimscapeComponentBlock  SourceFile=ResidentialPowerLoad  ComponentPath=ResidentialPowerLoad  ComponentVariants="[\"ResidentialPowerLoad\"]"  ComponentVariantNames="[\"ResidentialPowerLoad\"]"  ClassName=ResidentialPowerLoad  SchemaVersion=1  i_specify=off  i_priority=None  i=0 A  i_nominal_specify=off  i_nominal_unit=A  i_nominal_value=1  v_specify=off  v_priority=None  v=0 V  v_nominal_specify=off  v_nominal_unit=V  v_nominal_value=1
      settings: CopyFcn=simscape.engine.sli.internal.componentblockcallback(gcbh,'COPY')  PreCopyFcn=simscape.engine.sli.internal.componentblockcallback(gcbh,'PRECOPY')  PreDeleteFcn=simscape.engine.sli.internal.componentblockcallback(gcbh,'PREDELETE')  InternalSimscapePortConfiguration="{\"Bottom\":[],\"Left\":[{\"id\":\"Power\",\"label\":\"P\",\"type\":\"input\"},{\"id\":\"p\",\"label\":\"+\",\"type\":\"foundation.electrical.electrical\"}],\"Right\":[{\"id\":\"n\",\"label\":\"-\",\"type\":\"foundation.electrical.electrical\"}],\"Top\":[]}"
      mask Type: ResidentialPowerLoad
      mask Display: color('red');plot([0 1 1 0 0],[0 0 1 1 0]);plot([0.7,1],[1,0.7]);plot(-2,-1.75);plot(3, 1);disp('\n.ssc\nUnresolved')
  Simscape Bus1 : SimscapeBus  HierarchyStrings=High;Low
  Simulink-PS Converter : nesl_utility/Simulink-PS Converter  PhysicalDomain=network_engine_domain  SubClassName=ps_input  LeftPortType=input  RightPortType=output  PseudoPeriodic=off  Frequencies=[]  NoiseDistribution=none  NoiseParameters=[]  Unit=1  AffineConversion=off  FilteringAndDerivatives=provide  SimscapeFilterOrder=1  InputFilterTimeConstant=0.001  UdotUserProvided=0
  Terminator : Terminator
  Voltage Sensor : fl_lib/Electrical/Electrical Sensors/Voltage Sensor
  ResidentialOut : PMIOPort  Side=Right
  wires:
  "Residential power "/1 -> Simulink-PS Converter/1
  PS-Simulink Converter/1 -> Product/2  "voltage"
  PS-Simulink Converter1/1 -> Product/1  "current"
  Product/1 -> Terminator/1  "power"
  connections:
  Voltage Sensor/RConn2 -- Simscape Bus1/LConn2 -- Simscape Component/RConn1
  ResidentialOut/RConn1 -- Simscape Bus1/RConn1
  Simscape Component/LConn2 -- Current Sensor/RConn2 -- Voltage Sensor/LConn1
  Voltage Sensor/RConn1 -- PS-Simulink Converter/LConn1
  Simulink-PS Converter/RConn1 -- Simscape Component/LConn1
  Current Sensor/LConn1 -- Simscape Bus1/LConn1
  Current Sensor/RConn1 -- PS-Simulink Converter1/LConn1

== system T2_DCACpart_solar/Household 4 ==
  Current Sensor : fl_lib/Electrical/Electrical Sensors/Current Sensor
  PS-Simulink Converter : nesl_utility/PS-Simulink Converter  PhysicalDomain=network_engine_domain  SubClassName=ps_output  LeftPortType=input  RightPortType=output  PseudoPeriodic=off  Frequencies=[]  VectorFormat=inherit  Unit=inherit  AffineConversion=off
  PS-Simulink Converter1 : nesl_utility/PS-Simulink Converter  PhysicalDomain=network_engine_domain  SubClassName=ps_output  LeftPortType=input  RightPortType=output  PseudoPeriodic=off  Frequencies=[]  VectorFormat=inherit  Unit=inherit  AffineConversion=off
  Product : Product
  "Residential power " : simulink/Sources/Repeating Sequence Interpolated  OutValues=[2.8 2.5 2 2 2.2 2.5 2.8 3.4 3.6 3.8 4 4 4 4 4 4 4 4 4 4 3.8 3.5 3.2 3]*1000  TimeValues=[0 1 2 3 4 5 6 7 8 9 10 11 12 13 14 15 16 17 18 19 20 21 22 23]  LookUpMeth=Interpolation-Use End Values  tsamp=1e-4  OutMin=[]  OutMax=[]  OutDataTypeStr=double  OutputDataTypeScalingMode=double  OutDataType=fixdt(0,8)  OutScaling=2^-10
  Simscape Component : SimscapeComponentBlock  SourceFile=ResidentialPowerLoad  ComponentPath=ResidentialPowerLoad  ComponentVariants="[\"ResidentialPowerLoad\"]"  ComponentVariantNames="[\"ResidentialPowerLoad\"]"  ClassName=ResidentialPowerLoad  SchemaVersion=1  i_specify=off  i_priority=None  i=0 A  i_nominal_specify=off  i_nominal_unit=A  i_nominal_value=1  v_specify=off  v_priority=None  v=0 V  v_nominal_specify=off  v_nominal_unit=V  v_nominal_value=1
      settings: CopyFcn=simscape.engine.sli.internal.componentblockcallback(gcbh,'COPY')  PreCopyFcn=simscape.engine.sli.internal.componentblockcallback(gcbh,'PRECOPY')  PreDeleteFcn=simscape.engine.sli.internal.componentblockcallback(gcbh,'PREDELETE')  InternalSimscapePortConfiguration="{\"Bottom\":[],\"Left\":[{\"id\":\"Power\",\"label\":\"P\",\"type\":\"input\"},{\"id\":\"p\",\"label\":\"+\",\"type\":\"foundation.electrical.electrical\"}],\"Right\":[{\"id\":\"n\",\"label\":\"-\",\"type\":\"foundation.electrical.electrical\"}],\"Top\":[]}"
      mask Type: ResidentialPowerLoad
      mask Display: color('red');plot([0 1 1 0 0],[0 0 1 1 0]);plot([0.7,1],[1,0.7]);plot(-2,-1.75);plot(3, 1);disp('\n.ssc\nUnresolved')
  Simscape Bus1 : SimscapeBus  HierarchyStrings=High;Low
  Simulink-PS Converter : nesl_utility/Simulink-PS Converter  PhysicalDomain=network_engine_domain  SubClassName=ps_input  LeftPortType=input  RightPortType=output  PseudoPeriodic=off  Frequencies=[]  NoiseDistribution=none  NoiseParameters=[]  Unit=1  AffineConversion=off  FilteringAndDerivatives=provide  SimscapeFilterOrder=1  InputFilterTimeConstant=0.001  UdotUserProvided=0
  Terminator : Terminator
  Voltage Sensor : fl_lib/Electrical/Electrical Sensors/Voltage Sensor
  ResidentialOut : PMIOPort  Side=Right
  wires:
  Product/1 -> Terminator/1  "power"
  PS-Simulink Converter1/1 -> Product/1  "current"
  PS-Simulink Converter/1 -> Product/2  "voltage"
  "Residential power "/1 -> Simulink-PS Converter/1
  connections:
  Current Sensor/RConn1 -- PS-Simulink Converter1/LConn1
  Current Sensor/LConn1 -- Simscape Bus1/LConn1
  Simulink-PS Converter/RConn1 -- Simscape Component/LConn1
  Voltage Sensor/RConn1 -- PS-Simulink Converter/LConn1
  Voltage Sensor/LConn1 -- Current Sensor/RConn2 -- Simscape Component/LConn2
  ResidentialOut/RConn1 -- Simscape Bus1/RConn1
  Simscape Component/RConn1 -- Simscape Bus1/LConn2 -- Voltage Sensor/RConn2

== system T2_DCACpart_solar/Household 5 ==
  Current Sensor : fl_lib/Electrical/Electrical Sensors/Current Sensor
  PS-Simulink Converter : nesl_utility/PS-Simulink Converter  PhysicalDomain=network_engine_domain  SubClassName=ps_output  LeftPortType=input  RightPortType=output  PseudoPeriodic=off  Frequencies=[]  VectorFormat=inherit  Unit=inherit  AffineConversion=off
  PS-Simulink Converter1 : nesl_utility/PS-Simulink Converter  PhysicalDomain=network_engine_domain  SubClassName=ps_output  LeftPortType=input  RightPortType=output  PseudoPeriodic=off  Frequencies=[]  VectorFormat=inherit  Unit=inherit  AffineConversion=off
  Product : Product
  "Residential power " : simulink/Sources/Repeating Sequence Interpolated  OutValues=[2.8 2.5 2 2 2.2 2.5 2.8 3.4 3.6 3.8 4 4 4 4 4 4 4 4 4 4 3.8 3.5 3.2 3]*1000  TimeValues=[0 1 2 3 4 5 6 7 8 9 10 11 12 13 14 15 16 17 18 19 20 21 22 23]  LookUpMeth=Interpolation-Use End Values  tsamp=1e-4  OutMin=[]  OutMax=[]  OutDataTypeStr=double  OutputDataTypeScalingMode=double  OutDataType=fixdt(0,8)  OutScaling=2^-10
  Simscape Component : SimscapeComponentBlock  SourceFile=ResidentialPowerLoad  ComponentPath=ResidentialPowerLoad  ComponentVariants="[\"ResidentialPowerLoad\"]"  ComponentVariantNames="[\"ResidentialPowerLoad\"]"  ClassName=ResidentialPowerLoad  SchemaVersion=1  i_specify=off  i_priority=None  i=0 A  i_nominal_specify=off  i_nominal_unit=A  i_nominal_value=1  v_specify=off  v_priority=None  v=0 V  v_nominal_specify=off  v_nominal_unit=V  v_nominal_value=1
      settings: CopyFcn=simscape.engine.sli.internal.componentblockcallback(gcbh,'COPY')  PreCopyFcn=simscape.engine.sli.internal.componentblockcallback(gcbh,'PRECOPY')  PreDeleteFcn=simscape.engine.sli.internal.componentblockcallback(gcbh,'PREDELETE')  InternalSimscapePortConfiguration="{\"Bottom\":[],\"Left\":[{\"id\":\"Power\",\"label\":\"P\",\"type\":\"input\"},{\"id\":\"p\",\"label\":\"+\",\"type\":\"foundation.electrical.electrical\"}],\"Right\":[{\"id\":\"n\",\"label\":\"-\",\"type\":\"foundation.electrical.electrical\"}],\"Top\":[]}"
      mask Type: ResidentialPowerLoad
      mask Display: color('red');plot([0 1 1 0 0],[0 0 1 1 0]);plot([0.7,1],[1,0.7]);plot(-2,-1.75);plot(3, 1);disp('\n.ssc\nUnresolved')
  Simscape Bus1 : SimscapeBus  HierarchyStrings=High;Low
  Simulink-PS Converter : nesl_utility/Simulink-PS Converter  PhysicalDomain=network_engine_domain  SubClassName=ps_input  LeftPortType=input  RightPortType=output  PseudoPeriodic=off  Frequencies=[]  NoiseDistribution=none  NoiseParameters=[]  Unit=1  AffineConversion=off  FilteringAndDerivatives=provide  SimscapeFilterOrder=1  InputFilterTimeConstant=0.001  UdotUserProvided=0
  Terminator : Terminator
  Voltage Sensor : fl_lib/Electrical/Electrical Sensors/Voltage Sensor
  ResidentialOut : PMIOPort  Side=Right
  wires:
  "Residential power "/1 -> Simulink-PS Converter/1
  PS-Simulink Converter/1 -> Product/2  "voltage"
  PS-Simulink Converter1/1 -> Product/1  "current"
  Product/1 -> Terminator/1  "power"
  connections:
  Voltage Sensor/RConn2 -- Simscape Bus1/LConn2 -- Simscape Component/RConn1
  ResidentialOut/RConn1 -- Simscape Bus1/RConn1
  Simscape Component/LConn2 -- Current Sensor/RConn2 -- Voltage Sensor/LConn1
  Voltage Sensor/RConn1 -- PS-Simulink Converter/LConn1
  Simulink-PS Converter/RConn1 -- Simscape Component/LConn1
  Current Sensor/LConn1 -- Simscape Bus1/LConn1
  Current Sensor/RConn1 -- PS-Simulink Converter1/LConn1

== system T2_DCACpart_solar/Household 6 ==
  Current Sensor : fl_lib/Electrical/Electrical Sensors/Current Sensor
  PS-Simulink Converter : nesl_utility/PS-Simulink Converter  PhysicalDomain=network_engine_domain  SubClassName=ps_output  LeftPortType=input  RightPortType=output  PseudoPeriodic=off  Frequencies=[]  VectorFormat=inherit  Unit=inherit  AffineConversion=off
  PS-Simulink Converter1 : nesl_utility/PS-Simulink Converter  PhysicalDomain=network_engine_domain  SubClassName=ps_output  LeftPortType=input  RightPortType=output  PseudoPeriodic=off  Frequencies=[]  VectorFormat=inherit  Unit=inherit  AffineConversion=off
  Product : Product
  "Residential power " : simulink/Sources/Repeating Sequence Interpolated  OutValues=[2.8 2.5 2 2 2.2 2.5 2.8 3.4 3.6 3.8 4 4 4 4 4 4 4 4 4 4 3.8 3.5 3.2 3]*1000  TimeValues=[0 1 2 3 4 5 6 7 8 9 10 11 12 13 14 15 16 17 18 19 20 21 22 23]  LookUpMeth=Interpolation-Use End Values  tsamp=1e-4  OutMin=[]  OutMax=[]  OutDataTypeStr=double  OutputDataTypeScalingMode=double  OutDataType=fixdt(0,8)  OutScaling=2^-10
  Simscape Component : SimscapeComponentBlock  SourceFile=ResidentialPowerLoad  ComponentPath=ResidentialPowerLoad  ComponentVariants="[\"ResidentialPowerLoad\"]"  ComponentVariantNames="[\"ResidentialPowerLoad\"]"  ClassName=ResidentialPowerLoad  SchemaVersion=1  i_specify=off  i_priority=None  i=0 A  i_nominal_specify=off  i_nominal_unit=A  i_nominal_value=1  v_specify=off  v_priority=None  v=0 V  v_nominal_specify=off  v_nominal_unit=V  v_nominal_value=1
      settings: CopyFcn=simscape.engine.sli.internal.componentblockcallback(gcbh,'COPY')  PreCopyFcn=simscape.engine.sli.internal.componentblockcallback(gcbh,'PRECOPY')  PreDeleteFcn=simscape.engine.sli.internal.componentblockcallback(gcbh,'PREDELETE')  InternalSimscapePortConfiguration="{\"Bottom\":[],\"Left\":[{\"id\":\"Power\",\"label\":\"P\",\"type\":\"input\"},{\"id\":\"p\",\"label\":\"+\",\"type\":\"foundation.electrical.electrical\"}],\"Right\":[{\"id\":\"n\",\"label\":\"-\",\"type\":\"foundation.electrical.electrical\"}],\"Top\":[]}"
      mask Type: ResidentialPowerLoad
      mask Display: color('red');plot([0 1 1 0 0],[0 0 1 1 0]);plot([0.7,1],[1,0.7]);plot(-2,-1.75);plot(3, 1);disp('\n.ssc\nUnresolved')
  Simscape Bus1 : SimscapeBus  HierarchyStrings=High;Low
  Simulink-PS Converter : nesl_utility/Simulink-PS Converter  PhysicalDomain=network_engine_domain  SubClassName=ps_input  LeftPortType=input  RightPortType=output  PseudoPeriodic=off  Frequencies=[]  NoiseDistribution=none  NoiseParameters=[]  Unit=1  AffineConversion=off  FilteringAndDerivatives=provide  SimscapeFilterOrder=1  InputFilterTimeConstant=0.001  UdotUserProvided=0
  Terminator : Terminator
  Voltage Sensor : fl_lib/Electrical/Electrical Sensors/Voltage Sensor
  ResidentialOut : PMIOPort  Side=Right
  wires:
  Product/1 -> Terminator/1  "power"
  PS-Simulink Converter1/1 -> Product/1  "current"
  PS-Simulink Converter/1 -> Product/2  "voltage"
  "Residential power "/1 -> Simulink-PS Converter/1
  connections:
  Current Sensor/RConn1 -- PS-Simulink Converter1/LConn1
  Current Sensor/LConn1 -- Simscape Bus1/LConn1
  Simulink-PS Converter/RConn1 -- Simscape Component/LConn1
  Voltage Sensor/RConn1 -- PS-Simulink Converter/LConn1
  Voltage Sensor/LConn1 -- Current Sensor/RConn2 -- Simscape Component/LConn2
  ResidentialOut/RConn1 -- Simscape Bus1/RConn1
  Simscape Component/RConn1 -- Simscape Bus1/LConn2 -- Voltage Sensor/RConn2

== system T2_DCACpart_solar/Household 7 ==
  Current Sensor : fl_lib/Electrical/Electrical Sensors/Current Sensor
  PS-Simulink Converter : nesl_utility/PS-Simulink Converter  PhysicalDomain=network_engine_domain  SubClassName=ps_output  LeftPortType=input  RightPortType=output  PseudoPeriodic=off  Frequencies=[]  VectorFormat=inherit  Unit=inherit  AffineConversion=off
  PS-Simulink Converter1 : nesl_utility/PS-Simulink Converter  PhysicalDomain=network_engine_domain  SubClassName=ps_output  LeftPortType=input  RightPortType=output  PseudoPeriodic=off  Frequencies=[]  VectorFormat=inherit  Unit=inherit  AffineConversion=off
  Product : Product
  "Residential power " : simulink/Sources/Repeating Sequence Interpolated  OutValues=[2.8 2.5 2 2 2.2 2.5 2.8 3.4 3.6 3.8 4 4 4 4 4 4 4 4 4 4 3.8 3.5 3.2 3]*1000  TimeValues=[0 1 2 3 4 5 6 7 8 9 10 11 12 13 14 15 16 17 18 19 20 21 22 23]  LookUpMeth=Interpolation-Use End Values  tsamp=1e-4  OutMin=[]  OutMax=[]  OutDataTypeStr=double  OutputDataTypeScalingMode=double  OutDataType=fixdt(0,8)  OutScaling=2^-10
  Simscape Component : SimscapeComponentBlock  SourceFile=ResidentialPowerLoad  ComponentPath=ResidentialPowerLoad  ComponentVariants="[\"ResidentialPowerLoad\"]"  ComponentVariantNames="[\"ResidentialPowerLoad\"]"  ClassName=ResidentialPowerLoad  SchemaVersion=1  i_specify=off  i_priority=None  i=0 A  i_nominal_specify=off  i_nominal_unit=A  i_nominal_value=1  v_specify=off  v_priority=None  v=0 V  v_nominal_specify=off  v_nominal_unit=V  v_nominal_value=1
      settings: CopyFcn=simscape.engine.sli.internal.componentblockcallback(gcbh,'COPY')  PreCopyFcn=simscape.engine.sli.internal.componentblockcallback(gcbh,'PRECOPY')  PreDeleteFcn=simscape.engine.sli.internal.componentblockcallback(gcbh,'PREDELETE')  InternalSimscapePortConfiguration="{\"Bottom\":[],\"Left\":[{\"id\":\"Power\",\"label\":\"P\",\"type\":\"input\"},{\"id\":\"p\",\"label\":\"+\",\"type\":\"foundation.electrical.electrical\"}],\"Right\":[{\"id\":\"n\",\"label\":\"-\",\"type\":\"foundation.electrical.electrical\"}],\"Top\":[]}"
      mask Type: ResidentialPowerLoad
      mask Display: color('red');plot([0 1 1 0 0],[0 0 1 1 0]);plot([0.7,1],[1,0.7]);plot(-2,-1.75);plot(3, 1);disp('\n.ssc\nUnresolved')
  Simscape Bus1 : SimscapeBus  HierarchyStrings=High;Low
  Simulink-PS Converter : nesl_utility/Simulink-PS Converter  PhysicalDomain=network_engine_domain  SubClassName=ps_input  LeftPortType=input  RightPortType=output  PseudoPeriodic=off  Frequencies=[]  NoiseDistribution=none  NoiseParameters=[]  Unit=1  AffineConversion=off  FilteringAndDerivatives=provide  SimscapeFilterOrder=1  InputFilterTimeConstant=0.001  UdotUserProvided=0
  Terminator : Terminator
  Voltage Sensor : fl_lib/Electrical/Electrical Sensors/Voltage Sensor
  ResidentialOut : PMIOPort  Side=Right
  wires:
  Product/1 -> Terminator/1  "power"
  PS-Simulink Converter1/1 -> Product/1  "current"
  PS-Simulink Converter/1 -> Product/2  "voltage"
  "Residential power "/1 -> Simulink-PS Converter/1
  connections:
  Current Sensor/RConn1 -- PS-Simulink Converter1/LConn1
  Current Sensor/LConn1 -- Simscape Bus1/LConn1
  Simulink-PS Converter/RConn1 -- Simscape Component/LConn1
  Voltage Sensor/RConn1 -- PS-Simulink Converter/LConn1
  Voltage Sensor/LConn1 -- Current Sensor/RConn2 -- Simscape Component/LConn2
  ResidentialOut/RConn1 -- Simscape Bus1/RConn1
  Simscape Component/RConn1 -- Simscape Bus1/LConn2 -- Voltage Sensor/RConn2

== system T2_DCACpart_solar/Household 8 ==
  Current Sensor : fl_lib/Electrical/Electrical Sensors/Current Sensor
  PS-Simulink Converter : nesl_utility/PS-Simulink Converter  PhysicalDomain=network_engine_domain  SubClassName=ps_output  LeftPortType=input  RightPortType=output  PseudoPeriodic=off  Frequencies=[]  VectorFormat=inherit  Unit=inherit  AffineConversion=off
  PS-Simulink Converter1 : nesl_utility/PS-Simulink Converter  PhysicalDomain=network_engine_domain  SubClassName=ps_output  LeftPortType=input  RightPortType=output  PseudoPeriodic=off  Frequencies=[]  VectorFormat=inherit  Unit=inherit  AffineConversion=off
  Product : Product
  "Residential power " : simulink/Sources/Repeating Sequence Interpolated  OutValues=[2.8 2.5 2 2 2.2 2.5 2.8 3.4 3.6 3.8 4 4 4 4 4 4 4 4 4 4 3.8 3.5 3.2 3]*1000  TimeValues=[0 1 2 3 4 5 6 7 8 9 10 11 12 13 14 15 16 17 18 19 20 21 22 23]  LookUpMeth=Interpolation-Use End Values  tsamp=1e-4  OutMin=[]  OutMax=[]  OutDataTypeStr=double  OutputDataTypeScalingMode=double  OutDataType=fixdt(0,8)  OutScaling=2^-10
  Simscape Component : SimscapeComponentBlock  SourceFile=ResidentialPowerLoad  ComponentPath=ResidentialPowerLoad  ComponentVariants="[\"ResidentialPowerLoad\"]"  ComponentVariantNames="[\"ResidentialPowerLoad\"]"  ClassName=ResidentialPowerLoad  SchemaVersion=1  i_specify=off  i_priority=None  i=0 A  i_nominal_specify=off  i_nominal_unit=A  i_nominal_value=1  v_specify=off  v_priority=None  v=0 V  v_nominal_specify=off  v_nominal_unit=V  v_nominal_value=1
      settings: CopyFcn=simscape.engine.sli.internal.componentblockcallback(gcbh,'COPY')  PreCopyFcn=simscape.engine.sli.internal.componentblockcallback(gcbh,'PRECOPY')  PreDeleteFcn=simscape.engine.sli.internal.componentblockcallback(gcbh,'PREDELETE')  InternalSimscapePortConfiguration="{\"Bottom\":[],\"Left\":[{\"id\":\"Power\",\"label\":\"P\",\"type\":\"input\"},{\"id\":\"p\",\"label\":\"+\",\"type\":\"foundation.electrical.electrical\"}],\"Right\":[{\"id\":\"n\",\"label\":\"-\",\"type\":\"foundation.electrical.electrical\"}],\"Top\":[]}"
      mask Type: ResidentialPowerLoad
      mask Display: color('red');plot([0 1 1 0 0],[0 0 1 1 0]);plot([0.7,1],[1,0.7]);plot(-2,-1.75);plot(3, 1);disp('\n.ssc\nUnresolved')
  Simscape Bus1 : SimscapeBus  HierarchyStrings=High;Low
  Simulink-PS Converter : nesl_utility/Simulink-PS Converter  PhysicalDomain=network_engine_domain  SubClassName=ps_input  LeftPortType=input  RightPortType=output  PseudoPeriodic=off  Frequencies=[]  NoiseDistribution=none  NoiseParameters=[]  Unit=1  AffineConversion=off  FilteringAndDerivatives=provide  SimscapeFilterOrder=1  InputFilterTimeConstant=0.001  UdotUserProvided=0
  Terminator : Terminator
  Voltage Sensor : fl_lib/Electrical/Electrical Sensors/Voltage Sensor
  ResidentialOut : PMIOPort  Side=Right
  wires:
  "Residential power "/1 -> Simulink-PS Converter/1
  PS-Simulink Converter/1 -> Product/2  "voltage"
  PS-Simulink Converter1/1 -> Product/1  "current"
  Product/1 -> Terminator/1  "power"
  connections:
  Voltage Sensor/RConn2 -- Simscape Bus1/LConn2 -- Simscape Component/RConn1
  ResidentialOut/RConn1 -- Simscape Bus1/RConn1
  Simscape Component/LConn2 -- Current Sensor/RConn2 -- Voltage Sensor/LConn1
  Voltage Sensor/RConn1 -- PS-Simulink Converter/LConn1
  Simulink-PS Converter/RConn1 -- Simscape Component/LConn1
  Current Sensor/LConn1 -- Simscape Bus1/LConn1
  Current Sensor/RConn1 -- PS-Simulink Converter1/LConn1
